simulink model "InvertedPendulum"  (R2017a)
settings: Solver=ode23s  StartTime=0.0  StopTime=100.0  RelTol=1e-3
values from neighbouring files (symbols this model uses):
  bth = 0.035    [InvertedPendulum_simulation.m]    (also in nonlinear_equations.m)
  bx = 4.900    (= 4.9)    [InvertedPendulum_simulation.m]    (also in nonlinear_equations.m)
  g = 9.806    [InvertedPendulum_simulation.m]    (also in linear_CartPend.m; nonlinear_equations.m; solving_equations.m = (m*L^2 + I)/alpha)
  I = 0.006    [InvertedPendulum_simulation.m]    (also in nonlinear_equations.m)
  L = 0.560    (= 0.56)    [InvertedPendulum_simulation.m]    (also in drawcartpend.m = 2; nonlinear_equations.m)
  m = 0.356    [InvertedPendulum_simulation.m]    (also in nonlinear_equations.m)
  M = 4.800    (= 4.8)    [InvertedPendulum_simulation.m]    (also in nonlinear_equations.m)
settings Model: Creator=eddardd  LastModifiedBy=eddardd

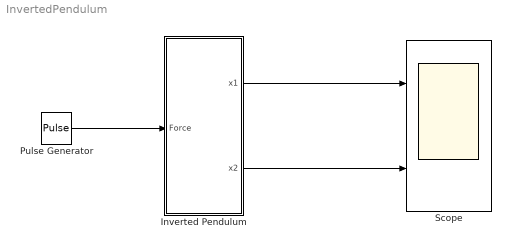
== system InvertedPendulum ==
  Inverted Pendulum : Subsystem
  Pulse Generator : DiscretePulseGenerator  PulseType=Time based  Period=10  PulseWidth=0.01
  Scope : Scope  NumInputPorts=2
  wires:
  Pulse Generator/1 -> Inverted Pendulum/1(Force)
  Inverted Pendulum/1(x1) -> Scope/1
  Inverted Pendulum/2(x2) -> Scope/2

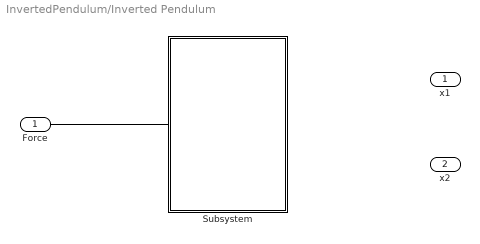
== system InvertedPendulum/Inverted Pendulum ==
  Force : Inport
  Subsystem : Subsystem
  x1 : Outport
  x2 : Outport  Port=2
  wires:
  Force/1 -> ?
  ? -> x1/1
  ? -> x2/1

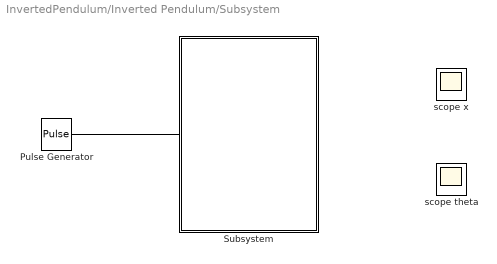
== system InvertedPendulum/Inverted Pendulum/Subsystem ==
  Pulse Generator : DiscretePulseGenerator  PulseType=Time based  Period=0.01  PulseWidth=5
  Subsystem : Subsystem
  scope theta : Scope
  scope x : Scope
  wires:
  ? -> scope x/1
  ? -> scope theta/1
  Pulse Generator/1 -> ?

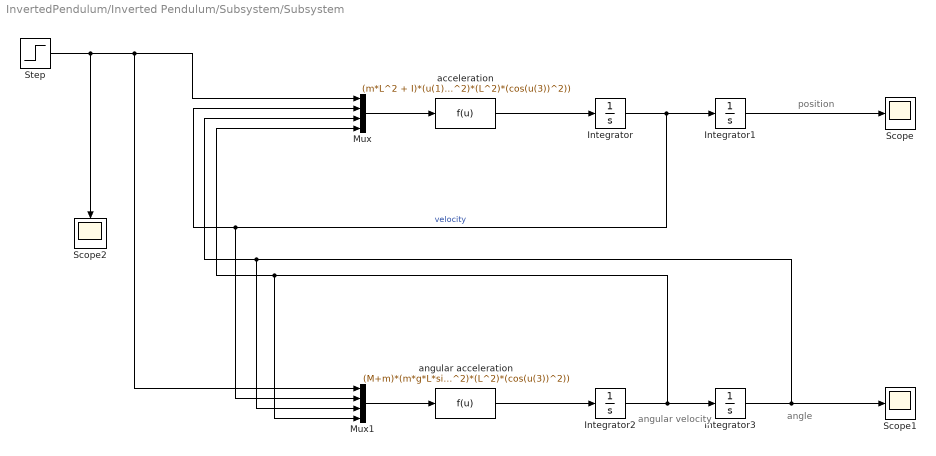
== system InvertedPendulum/Inverted Pendulum/Subsystem/Subsystem ==
  note: angle
  note: angular velocity
  note: position
  Integrator{,1..3} (4 alike) : Integrator
  Mux : Mux
  Mux1 : Mux
  Scope : Scope
  Scope1 : Scope
  Scope2 : Scope
  Step : Step  SampleTime=0
  acceleration : Fcn  Expr=(m*L^2 + I)*(u(1) - m * L * sin(u(3)) * u(4)^2 - bx * u(2)) + m * L * cos(u(3)) * (m*g*L*sin(u(3)) - bth * u(4))/((M+m)*(m*L^2 + I) - (m^2)*(L^2)*(cos(u(3))^2))
  angular acceleration : Fcn  Expr=(M+m)*(m*g*L*sin(u(3)) - bth * u(4)) + m * L * cos(u(3)) * (u(1) - m * L * (u(4)^2) * sin(u(3)) - bx * u(2)) / ((M+m)*(m*L^2 + I) - (m^2)*(L^2)*(cos(u(3))^2))
  wires:
  Step/1 -> Scope2/1, Mux1/1, Mux/1
  Mux1/1 -> angular acceleration/1
  angular acceleration/1 -> Integrator2/1
  Integrator2/1 -> Mux1/4, Mux/4, Integrator3/1
  Mux/1 -> acceleration/1
  acceleration/1 -> Integrator/1
  Integrator1/1 -> Scope/1
  Integrator/1 -> Mux1/2, Mux/2, Integrator1/1  "velocity"
  Integrator3/1 -> Scope1/1, Mux1/3, Mux/3
